simulink model "Complete_Model_with_simulation"  (R2014a)
settings: Solver=ode45  StartTime=0.0  StopTime=10.0  FixedStep=1  RelTol=1e-3
values from neighbouring files (symbols this model uses):
  C1 = (eff*K_m*K_g)/(R_a*J_eq)    (= 66.3942391304)    [Parameters.m]
  C2 = (B_eq/J_eq)+((eff*K_m*K_m*K_g*K_g)/(R_a*J_eq))    (= 37.3861974239)    [Parameters.m]
  K_d = 0.6987    [Parameters.m]
  K_d_x = 0.4985    [Parameters.m]
  K_p = 41.292    [Parameters.m]
  K_p_x = 0.87    [Parameters.m]
  L = 0.1675    [Parameters.m]
  r = 0.0254    [Parameters.m]
libraries: vrlib x4
settings Model: Creator=USER PC  LastModifiedBy=Khaled Hefnawy
settings DebuggingCC: MergeDetectMultiDrivingBlocksExec=error

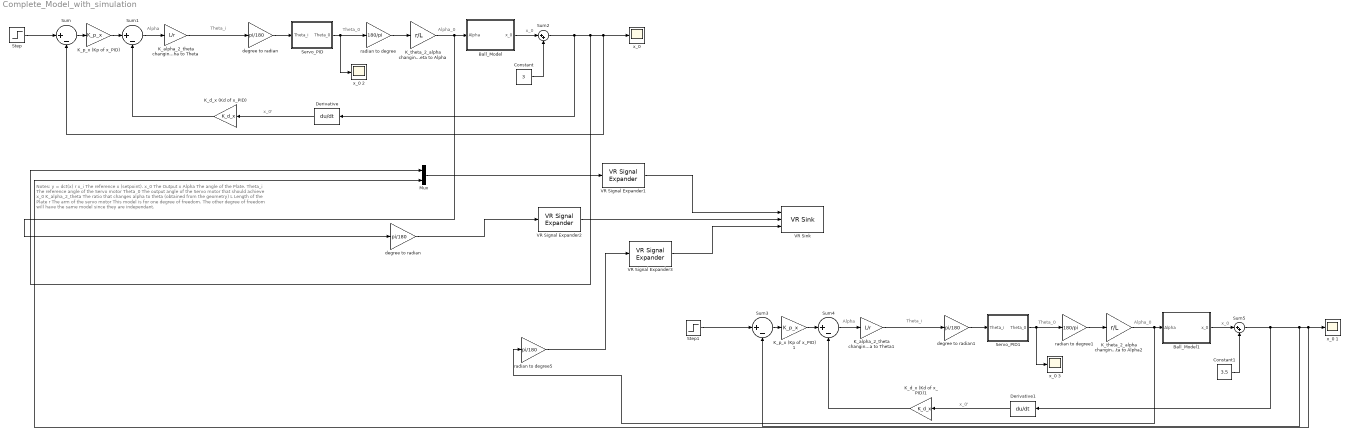
== system Complete_Model_with_simulation ==
  note: Notes: y = dct(x) r
      |
      | x_i The reference x (setpoint).
      | x_0 The Output x
      | Alpha The angle of the Plate.
      | Theta_i The reference angle of the Servo motor
      | Theta_0 The output angle of the Servo motor that should achieve x_0
      | K_alpha_2_theta The ratio that changes alpha to theta (obtained from the geometry)
      | L Length of the Plate
      | r The arm of the servo motor
      |
      | This model is for one degree of freedom. The other degree of freedom will have the same model since they are independant.
  note: x_0'
  note: x_0
  note: Alpha_0
  note: Theta_0
  note: Theta_i
  note: Alpha
  note: x_0'
  note: x_0
  note: Alpha_0
  note: Theta_0
  note: Theta_i
  note: Alpha
  Ball_Model : Subsystem
  Ball_Model1 : Subsystem
  Constant : Constant  Value=3
  Constant1 : Constant  Value=3.5
  Derivative : Derivative
  Derivative1 : Derivative
  K_alpha_2_theta changing Alpha to Theta : Gain  Gain=L/r
  K_alpha_2_theta changing Alpha to Theta1 : Gain  Gain=L/r
  K_d_x (Kd of x_PID) : Gain  Gain=K_d_x
  K_d_x (Kd of x_PID)1 : Gain  Gain=K_d_x
  "K_p_x (Kp of x_PID) " : Gain  Gain=K_p_x
  K_p_x (Kp of x_PID) 1 : Gain  Gain=K_p_x
  K_theta_2_alpha changing Theta to Alpha : Gain  Gain=r/L
  K_theta_2_alpha changing Theta to Alpha2 : Gain  Gain=r/L
  Mux : Mux  Inputs=2
  Servo_PID : Subsystem
  Servo_PID1 : Subsystem
  Step : Step  SampleTime=0
  Step1 : Step  After=2  SampleTime=0
  Sum{,1,3..4} (4 alike) : Sum  Inputs=|+-
  Sum2 : Sum  Inputs=|++
  Sum5 : Sum  Inputs=|++
  VR Signal Expander1 : vrlib/VR Signal Expander  outwidth=3  outidx=[1 3]
  VR Signal Expander2 : vrlib/VR Signal Expander  outwidth=4  outidx=[4]
  VR Signal Expander3 : vrlib/VR Signal Expander  outwidth=4  outidx=[4]
  VR Sink : vrlib/VR Sink  InstantiateOnLoad=on  SampleTime=0.01  ViewEnable=on  RemoteChange=off  RemoteView=off  FieldsWritten=Ball.translation.3.1.1.double#plateX.rotation.4.1.1.double#plateY.rotation.4.1.1.double  WorldFileName=C:\Users\Khaled Hefnawy\Desktop\bouncing_ball_3d\bouncing_ball_3d\ball_and_plate.wrl  AutoView=off  VideoDimensions=[]  AllowVariableSize=off
  degree to radian : Gain  Gain=pi/180
  "degree to radian " : Gain  Gain=pi/180
  degree to radian1 : Gain  Gain=pi/180
  radian to degree : Gain  Gain=180/pi
  radian to degree1 : Gain  Gain=180/pi
  radian to degree5 : Gain  Gain=pi/180
  x_0 {,1..3} (4 alike) : Scope
      x_0 2 settings: SaveName=ScopeData2
      x_0 3 settings: SaveName=ScopeData3
  wires:
  Sum/1 -> "K_p_x (Kp of x_PID) "/1
  "K_p_x (Kp of x_PID) "/1 -> Sum1/1
  K_d_x (Kd of x_PID)/1 -> Sum1/2
  Sum1/1 -> K_alpha_2_theta changing Alpha to Theta/1
  K_alpha_2_theta changing Alpha to Theta/1 -> degree to radian/1
  Derivative/1 -> K_d_x (Kd of x_PID)/1
  radian to degree/1 -> K_theta_2_alpha changing Theta to Alpha/1
  degree to radian/1 -> Servo_PID/1(Theta_i)
  Step/1 -> Sum/1
  Sum2/1 -> Derivative/1, Mux/1, Sum/2, "x_0 "/1
  Servo_PID/1(Theta_0) -> x_0 2/1, radian to degree/1
  Mux/1 -> VR Signal Expander1/1
  K_theta_2_alpha changing Theta to Alpha/1 -> "degree to radian "/1, Ball_Model/1(Alpha)
  Ball_Model/1("x_0 ") -> Sum2/1
  Constant/1 -> Sum2/2
  VR Signal Expander1/1 -> VR Sink/1
  Sum3/1 -> K_p_x (Kp of x_PID) 1/1
  K_p_x (Kp of x_PID) 1/1 -> Sum4/1
  K_d_x (Kd of x_PID)1/1 -> Sum4/2
  Sum4/1 -> K_alpha_2_theta changing Alpha to Theta1/1
  K_alpha_2_theta changing Alpha to Theta1/1 -> degree to radian1/1
  Derivative1/1 -> K_d_x (Kd of x_PID)1/1
  radian to degree1/1 -> K_theta_2_alpha changing Theta to Alpha2/1
  degree to radian1/1 -> Servo_PID1/1(Theta_i)
  Sum5/1 -> Derivative1/1, Sum3/2, Mux/2, x_0 1/1
  Servo_PID1/1(Theta_0) -> x_0 3/1, radian to degree1/1
  K_theta_2_alpha changing Theta to Alpha2/1 -> radian to degree5/1, Ball_Model1/1(Alpha)
  Ball_Model1/1("x_0 ") -> Sum5/1
  VR Signal Expander2/1 -> VR Sink/2
  VR Signal Expander3/1 -> VR Sink/3
  Step1/1 -> Sum3/1
  Constant1/1 -> Sum5/2
  "degree to radian "/1 -> VR Signal Expander2/1
  radian to degree5/1 -> VR Signal Expander3/1

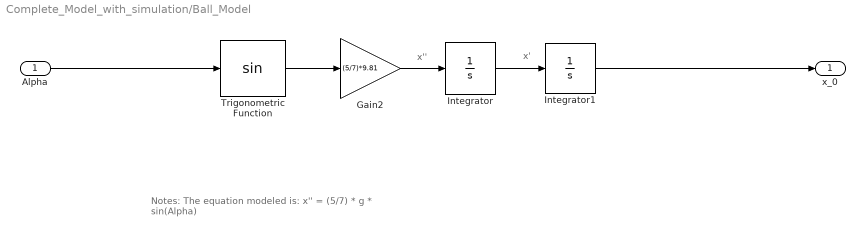
== system Complete_Model_with_simulation/Ball_Model ==
  note: Notes:
      |
      | The equation modeled is:
      |
      | x'' = (5/7) * g * sin(Alpha)
  note: x'
  note: x''
  Alpha : Inport
  Gain2 : Gain  Gain=(5/7)*9.81
  Integrator : Integrator
  Integrator1 : Integrator
  Trigonometric Function : Trigonometry
  "x_0 " : Outport
  wires:
  Integrator1/1 -> "x_0 "/1
  Gain2/1 -> Integrator/1
  Integrator/1 -> Integrator1/1
  Trigonometric Function/1 -> Gain2/1
  Alpha/1 -> Trigonometric Function/1

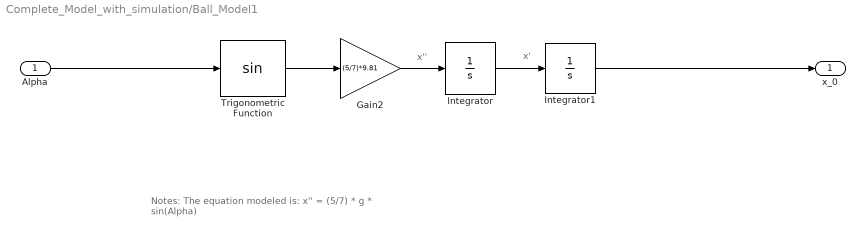
== system Complete_Model_with_simulation/Ball_Model1 ==
  note: Notes:
      |
      | The equation modeled is:
      |
      | x'' = (5/7) * g * sin(Alpha)
  note: x'
  note: x''
  Alpha : Inport
  Gain2 : Gain  Gain=(5/7)*9.81
  Integrator : Integrator
  Integrator1 : Integrator
  Trigonometric Function : Trigonometry
  "x_0 " : Outport
  wires:
  Integrator1/1 -> "x_0 "/1
  Gain2/1 -> Integrator/1
  Integrator/1 -> Integrator1/1
  Trigonometric Function/1 -> Gain2/1
  Alpha/1 -> Trigonometric Function/1

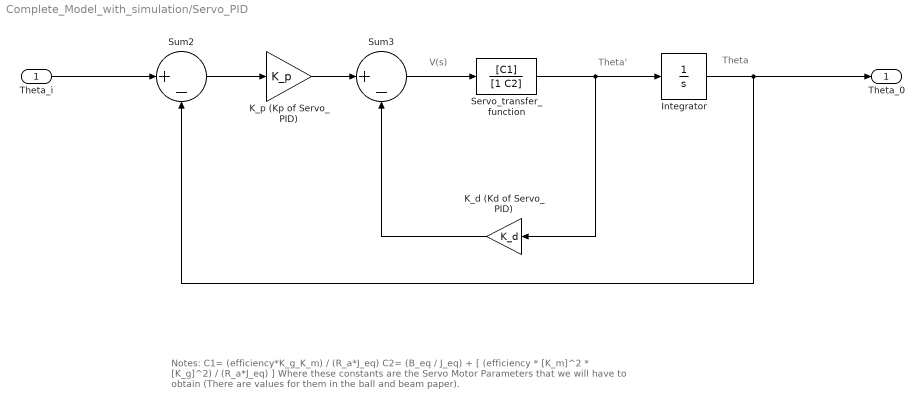
== system Complete_Model_with_simulation/Servo_PID ==
  note: Notes:
      |
      | C1= (efficiency*K_g_K_m) / (R_a*J_eq)
      | C2= (B_eq / J_eq) + [ (efficiency * [K_m]^2 * [K_g]^2) / (R_a*J_eq) ]
      |
      | Where these constants are the Servo Motor Parameters that we will have to obtain (There are values for them in the ball and beam paper).
  note: Theta
  note: Theta'
  note: V(s)
  Theta_i : Inport
  Integrator : Integrator
  K_d (Kd of Servo_PID) : Gain  Gain=K_d
  K_p (Kp of Servo_PID) : Gain  Gain=K_p
  "Servo_transfer_function " : TransferFcn  Numerator=[C1]  Denominator=[1 C2]
  Sum2 : Sum  Inputs=|+-
  Sum3 : Sum  Inputs=|+-
  Theta_0 : Outport
  wires:
  Theta_i/1 -> Sum2/1
  K_p (Kp of Servo_PID)/1 -> Sum3/1
  Sum2/1 -> K_p (Kp of Servo_PID)/1
  Integrator/1 -> Theta_0/1, Sum2/2
  K_d (Kd of Servo_PID)/1 -> Sum3/2
  Sum3/1 -> "Servo_transfer_function "/1
  "Servo_transfer_function "/1 -> K_d (Kd of Servo_PID)/1, Integrator/1

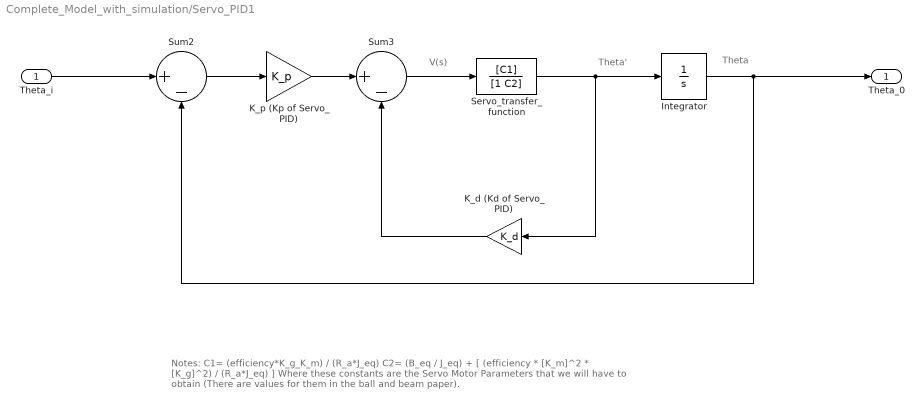
== system Complete_Model_with_simulation/Servo_PID1 ==
  note: Notes:
      |
      | C1= (efficiency*K_g_K_m) / (R_a*J_eq)
      | C2= (B_eq / J_eq) + [ (efficiency * [K_m]^2 * [K_g]^2) / (R_a*J_eq) ]
      |
      | Where these constants are the Servo Motor Parameters that we will have to obtain (There are values for them in the ball and beam paper).
  note: Theta
  note: Theta'
  note: V(s)
  Theta_i : Inport
  Integrator : Integrator
  K_d (Kd of Servo_PID) : Gain  Gain=K_d
  K_p (Kp of Servo_PID) : Gain  Gain=K_p
  "Servo_transfer_function " : TransferFcn  Numerator=[C1]  Denominator=[1 C2]
  Sum2 : Sum  Inputs=|+-
  Sum3 : Sum  Inputs=|+-
  Theta_0 : Outport
  wires:
  Theta_i/1 -> Sum2/1
  K_p (Kp of Servo_PID)/1 -> Sum3/1
  Sum2/1 -> K_p (Kp of Servo_PID)/1
  Integrator/1 -> Theta_0/1, Sum2/2
  K_d (Kd of Servo_PID)/1 -> Sum3/2
  Sum3/1 -> "Servo_transfer_function "/1
  "Servo_transfer_function "/1 -> K_d (Kd of Servo_PID)/1, Integrator/1
